simulink model "a1"  (R2024b)
settings: Solver=VariableStepAuto  StartTime=0.0  StopTime=10.0  RelTol=1e-3
values from neighbouring files (symbols this model uses):
  a = poly([-3, -3, -3])    [exam.m]    (also in exam2.m)
  p = [1; 1; 1]    [exam.m]    (also in exam3.m = [1; 0]; practical_exam_assignment3.m = [0, 1])
settings Model: Creator=lukiq  LastModifiedBy=lukiq

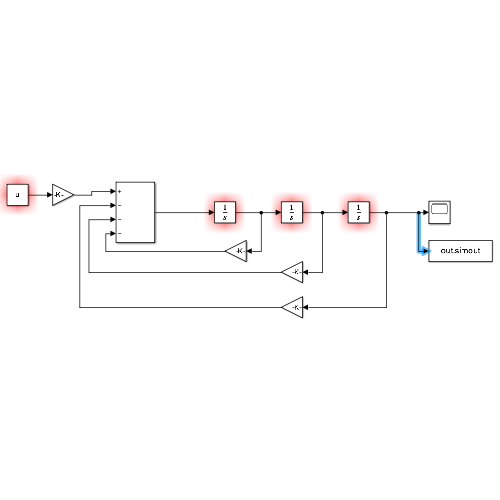
[thumbnail: Simulink's stored preview of the top-level diagram]
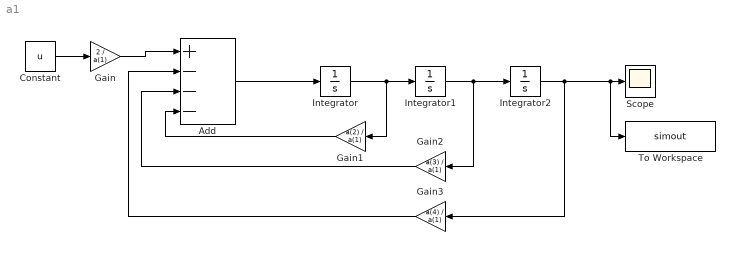
== system a1 ==
  Add : Sum  Inputs=+---
  Constant : Constant  Value=u
  Gain : Gain  Gain=2 / a(1)
  Gain1 : Gain  Gain=a(2) / a(1)
  Gain2 : Gain  Gain=a(3) / a(1)
  Gain3 : Gain  Gain=a(4) / a(1)
  Integrator : Integrator  InitialCondition=p(3)
  Integrator1 : Integrator  InitialCondition=p(2)
  Integrator2 : Integrator  InitialCondition=p(1)
  Scope : Scope
  To Workspace : ToWorkspace  VariableName=simout  SaveFormat=Timeseries  SampleTime=-1
  wires:
  Gain/1 -> Add/1
  Constant/1 -> Gain/1
  Add/1 -> Integrator/1
  Integrator/1 -> Gain1/1, Integrator1/1
  Integrator1/1 -> Gain2/1, Integrator2/1
  Integrator2/1 -> To Workspace/1, Scope/1, Gain3/1
  Gain1/1 -> Add/4
  Gain2/1 -> Add/3
  Gain3/1 -> Add/2
